simulink model "modelosMalhaAberta"  (R2021a)
settings: Solver=VariableStepAuto  StartTime=0.0  StopTime=4000  RelTol=1e-3
libraries: cstblocks x3
settings Model: SimulationMode=accelerator  Creator=pedroian  LastModifiedBy=pedroian

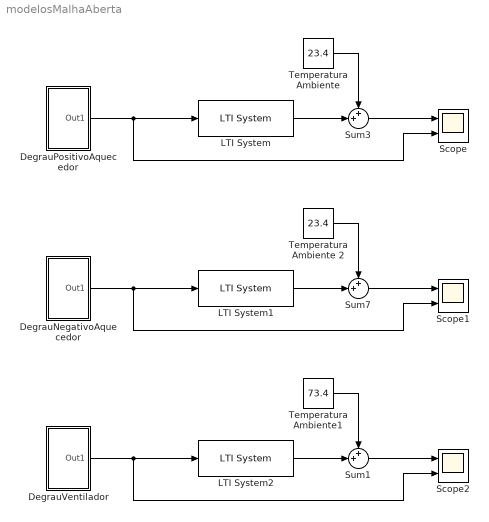
== system modelosMalhaAberta ==
  DegrauNegativoAquecedor : Subsystem
  DegrauPositivoAquecedor : Subsystem
  DegrauVentilador : Subsystem
  LTI System : cstblocks/LTI System  sys=tfAquecedorAquecimento  IC=[]
  LTI System1 : cstblocks/LTI System  sys=tfAquecedorResfriamento  IC=[]
  LTI System2 : cstblocks/LTI System  sys=tfVentiladorResfriamento  IC=[]
  Scope : Scope  NumInputPorts=2
  Scope1 : Scope  NumInputPorts=2
  Scope2 : Scope  NumInputPorts=2
  Sum1 : Sum  Inputs=++|
  Sum3 : Sum  Inputs=++|
  Sum7 : Sum  Inputs=++|
  Temperatura Ambiente : Constant  Value=23.4
  Temperatura Ambiente 2 : Constant  Value=23.4
  Temperatura Ambiente1 : Constant  Value=73.4
  wires:
  LTI System/1 -> Sum3/2
  Sum3/1 -> Scope/1
  Temperatura Ambiente/1 -> Sum3/1
  Sum7/1 -> Scope1/1
  Temperatura Ambiente 2/1 -> Sum7/1
  LTI System1/1 -> Sum7/2
  DegrauNegativoAquecedor/1(Out1) -> Scope1/2, LTI System1/1
  DegrauPositivoAquecedor/1(Out1) -> Scope/2, LTI System/1
  DegrauVentilador/1(Out1) -> Scope2/2, LTI System2/1
  LTI System2/1 -> Sum1/2
  Temperatura Ambiente1/1 -> Sum1/1
  Sum1/1 -> Scope2/1

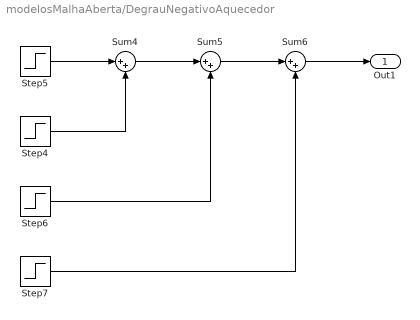
== system modelosMalhaAberta/DegrauNegativoAquecedor ==
  Step4 : Step  Time=2025  After=-25  SampleTime=0
  Step5 : Step  Time=1432  Before=100  After=75  SampleTime=0
  Step6 : Step  Time=2674  After=-25  SampleTime=0
  Step7 : Step  Time=3345  After=-25  SampleTime=0
  Sum4 : Sum  Inputs=|++
  Sum5 : Sum  Inputs=|++
  Sum6 : Sum  Inputs=|++
  Out1 : Outport
  wires:
  Sum4/1 -> Sum5/1
  Sum6/1 -> Out1/1
  Step7/1 -> Sum6/2
  Step6/1 -> Sum5/2
  Step4/1 -> Sum4/2
  Step5/1 -> Sum4/1
  Sum5/1 -> Sum6/1

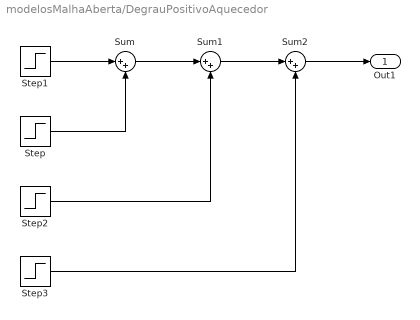
== system modelosMalhaAberta/DegrauPositivoAquecedor ==
  Step : Step  Time=399  After=25  SampleTime=0
  Step1 : Step  Time=84  After=25  SampleTime=0
  Step2 : Step  Time=844  After=25  SampleTime=0
  Step3 : Step  Time=1404  After=25  SampleTime=0
  Sum : Sum  Inputs=|++
  Sum1 : Sum  Inputs=|++
  Sum2 : Sum  Inputs=|++
  Out1 : Outport
  wires:
  Step2/1 -> Sum1/2
  Sum2/1 -> Out1/1
  Sum/1 -> Sum1/1
  Step/1 -> Sum/2
  Sum1/1 -> Sum2/1
  Step1/1 -> Sum/1
  Step3/1 -> Sum2/2

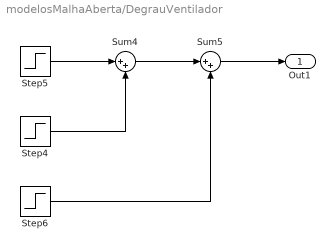
== system modelosMalhaAberta/DegrauVentilador ==
  Step4 : Step  Time=716  After=-500  SampleTime=0
  Step5 : Step  Time=448  After=500  SampleTime=0
  Step6 : Step  Time=997  After=1000  SampleTime=0
  Sum4 : Sum  Inputs=|++
  Sum5 : Sum  Inputs=|++
  Out1 : Outport
  wires:
  Sum4/1 -> Sum5/1
  Sum5/1 -> Out1/1
  Step6/1 -> Sum5/2
  Step4/1 -> Sum4/2
  Step5/1 -> Sum4/1
